simulink model "BOUCLE8VITESS2"  (R2014b)
settings: Solver=ode45  StartTime=0.0  StopTime=5.0  MaxStep=1e-5  MinStep=1e-7  RelTol=1e-3
undefined symbols (not defined in the file): D1, lagging, pulse
libraries: powerlib x9, powerlib_meascontrol x1, simulink x1
settings Model: Creator=Abdelhak  LastModifiedBy=Abdelhak

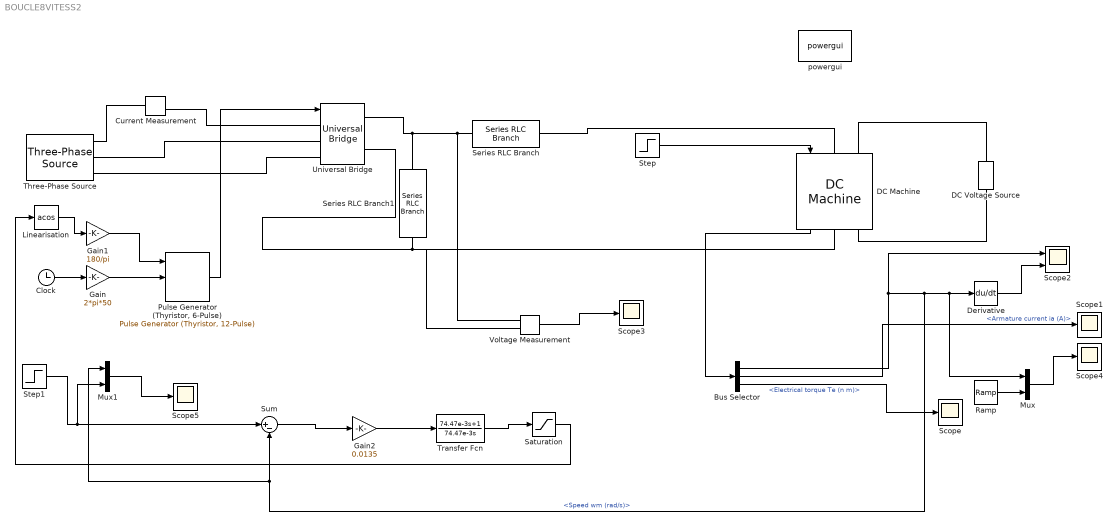
== system BOUCLE8VITESS2 ==
  Bus Selector : BusSelector  OutputSignals=Speed wm (rad/s),Armature current ia (A),Electrical torque Te (n m)
  Clock : Clock
  Current Measurement : powerlib/Measurements/Current Measurement  PhasorSimulation=off  OutputType=Complex  PSBequivalent=0
  DC Machine : powerlib/Machines/DC Machine  PresetModel=02: 5HP 240V 1750RPM Field:150V  MechanicalLoad=Torque TL  FieldType=Wound  ShowDetailedParameters=on  MeasurementBus=off  RLa=[0.78 0.016]  RLf=[150 112.5]  Laf=1.234  MachineConstant=Torque constant (N.m/A)  Ke=1.8  Kt=1.8  J=0.05  Bm=0.01  Tf=0  w0=1  Ifinit=1  TsPowergui=0  TsBlock=-1
  DC Voltage Source : powerlib/Electrical Sources/DC Voltage Source  Amplitude=150  Measurements=None
  Derivative : Derivative
  Gain : Gain  Gain=2*pi*50
  Gain1 : Gain  Gain=180/pi
  Gain2 : Gain  Gain=0.0135
  Linearisation : Trigonometry  Operator=acos
  Mux : Mux  Inputs=2
  Mux1 : Mux  Inputs=2
  "Pulse Generator (Thyristor, 6-Pulse)" : powerlib_meascontrol/Pulse & Signal Generators/Pulse Generator (Thyristor, 12-Pulse)  GenType=6-pulse  Delta=D1 (lagging)  pwidth=50  Double_Pulse=off  Ts=0
  Ramp : simulink/Sources/Ramp  slope=3195  start=0  X0=-21.18
  Saturation : Saturate  UpperLimit=1  LowerLimit=-1
  Scope{,1,3..5} (5 alike) : Scope
      Scope3 settings: SaveName=ScopeData3
      Scope4 settings: YMin=0  YMax=8000  SaveName=ScopeData4
      Scope5 settings: YMin=0  YMax=200  SaveName=ScopeData5
  Scope2 : Scope  NumInputPorts=2
      settings: YMin=0~-500  YMax=250~3500  SaveName=ScopeData2
  Series RLC Branch : powerlib/Elements/Series RLC Branch  LConnTagsString=__new0  RConnTagsString=__new0  BranchType=L  Resistance=1  Inductance=4e-3  SetiL0=off  InitialCurrent=0  Capacitance=1e-6  Setx0=off  InitialVoltage=0  Measurements=None
  Series RLC Branch1 : powerlib/Elements/Series RLC Branch  LConnTagsString=__new0  RConnTagsString=__new0  BranchType=C  Resistance=1  Inductance=1e-3  SetiL0=off  InitialCurrent=0  Capacitance=1e-5  Setx0=off  InitialVoltage=0  Measurements=None
  Step : Step  Time=3  After=10  SampleTime=0
  Step1 : Step  Time=3  Before=150  After=200  SampleTime=0
  Sum : Sum  Inputs=|+-
  Three-Phase Source : powerlib/Electrical Sources/Three-Phase Source  Voltage=220  PhaseAngle=0  Frequency=50  InternalConnection=Yg  SpecifyImpedance=off  Resistance=0.5  Inductance=0  ShortCircuitLevel=100e6  BaseVoltage=25e3  XRratio=7  BusType=swing  Pref=0  Qref=0  Qmin=-inf  Qmax=inf
  Transfer Fcn : TransferFcn  Numerator=[74.47e-3 1]  Denominator=[74.47e-3 0]
  Universal Bridge : powerlib/Power Electronics/Universal Bridge  Arms=3  SnubberResistance=1e5  SnubberCapacitance=inf  Device=Thyristors  Ron=1e-3  Lon=0  ForwardVoltages="[  0  0  ]"  ForwardVoltage=0  GTOparameters=[ 10e-6 , 20e-6 ]  IGBTparameters=[ 1e-6 , 2e-6 ]  Measurements=None  Measurements_2=None  converterType=Rectifier
  Voltage Measurement : powerlib/Measurements/Voltage Measurement  PhasorSimulation=off  OutputType=Complex  PSBequivalent=0
  powergui : powerlib/powergui  Priority=1  SimulationMode=Continuous  SolverType=Tustin/Backward Euler (TBE)  SampleTime=50e-6  frequency=60  SPID=off  DisableSnubberDevices=off  DisableRonSwitches=off  DisableVfSwitches=off  SwTol=0  DisplayEquations=off  Interpol=off  methode=off  Ts=100  frequencyindice=0  Pbase=100e6  ErrMax=1e-4  Iterations=50  UnitsV=kV  UnitsW=MW  FunctionMessages=off  echomessages=off  HookPort=off  EnableUseOfTLC=off  x0status=blocks  RestoreLinks=warning  ResistiveCurrentMeasurement=off  Frange=[0:2:500]  Ylog=off  Xlog=on  ShowGrid=off  save=off  variable=ZData  structure=0  ZoomFFT=off  StartTime=0.0  cycles=1  DisplayStyle=1  fundamental=60  FreqAxis=off  MaxFrequency=1000  frequencyindicesteady=1  RmsSteady=1  display=off
  wires:
  Step/1 -> DC Machine/1
  "Pulse Generator (Thyristor, 6-Pulse)"/1 -> Universal Bridge/1
  Gain/1 -> "Pulse Generator (Thyristor, 6-Pulse)"/2
  Clock/1 -> Gain/1
  DC Machine/1 -> Bus Selector/1
  Bus Selector/1 -> Mux1/1, Sum/2, Mux/1, Derivative/1, Scope2/1  "<Speed wm (rad/s)>"
  Bus Selector/2 -> Scope1/1  "<Armature current ia (A)>"
  Bus Selector/3 -> Scope/1  "<Electrical torque Te (n m)>"
  Gain1/1 -> "Pulse Generator (Thyristor, 6-Pulse)"/1
  Voltage Measurement/1 -> Scope3/1
  Linearisation/1 -> Gain1/1
  Derivative/1 -> Scope2/2
  Mux/1 -> Scope4/1
  Ramp/1 -> Mux/2
  Sum/1 -> Gain2/1
  Gain2/1 -> Transfer Fcn/1
  Transfer Fcn/1 -> Saturation/1
  Saturation/1 -> Linearisation/1
  Mux1/1 -> Scope5/1
  Step1/1 -> Sum/1, Mux1/2
  connections:
  DC Voltage Source/RConn1 -- DC Machine/LConn2
  DC Voltage Source/LConn1 -- DC Machine/RConn2
  Universal Bridge/RConn1 -- Series RLC Branch1/LConn1 -- Voltage Measurement/LConn1 -- Series RLC Branch/LConn1
  Universal Bridge/RConn2 -- Voltage Measurement/LConn2 -- DC Machine/RConn1 -- Series RLC Branch1/RConn1
  Three-Phase Source/RConn1 -- Current Measurement/LConn1
  Three-Phase Source/RConn3 -- Universal Bridge/LConn3
  Series RLC Branch/RConn1 -- DC Machine/LConn1
  Three-Phase Source/RConn2 -- Universal Bridge/LConn2
  Universal Bridge/LConn1 -- Current Measurement/RConn1
